simulink model "robo_stix_fn"  (Simulink 7.1)
settings: Solver=FixedStepDiscrete  StartTime=0.0  StopTime=10.0  RelTol=1e-3
settings Model: Creator=jporter  LastModifiedBy=jporter

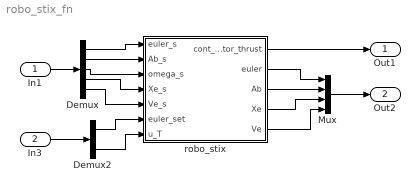
== system robo_stix_fn ==
  In1 : Inport  OutDataType=sfix(16)  OutScaling=2^0
  In3 : Inport  Port=2  OutDataType=sfix(16)  OutScaling=2^0
  Demux : Demux  Outputs=5
  Demux2 : Demux  Outputs=2
  Mux : Mux
  robo_stix : Subsystem
  Out1 : Outport  OutDataType=sfix(16)  OutScaling=2^0
  Out2 : Outport  Port=2  OutDataType=sfix(16)  OutScaling=2^0
  wires:
  Demux/1 -> robo_stix/1(euler_s)
  Demux/2 -> robo_stix/2(Ab_s)
  Demux/3 -> robo_stix/3(omega_s)
  Demux2/1 -> robo_stix/6(euler_set)
  Demux2/2 -> robo_stix/7(u_T)
  In1/1 -> Demux/1
  In3/1 -> Demux2/1
  robo_stix/1(cont_motor_thrust) -> Out1/1
  Mux/1 -> Out2/1
  robo_stix/2(euler) -> Mux/1
  robo_stix/3(Ab) -> Mux/2
  robo_stix/4(Xe) -> Mux/3
  robo_stix/5(Ve) -> Mux/4
  Demux/4 -> robo_stix/4(Xe_s)
  Demux/5 -> robo_stix/5(Ve_s)

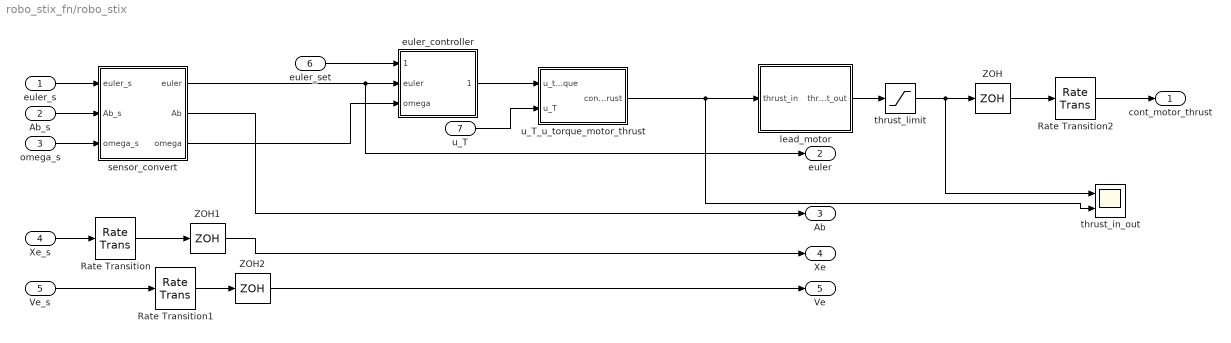
== system robo_stix_fn/robo_stix ==
  euler_s : Inport
  Ab_s : Inport  Port=2
  omega_s : Inport  Port=3
  Xe_s : Inport  Port=4
  Ve_s : Inport  Port=5
  euler_set : Inport  Port=6
  u_T : Inport  Port=7
  Rate Transition : RateTransition
  Rate Transition1 : RateTransition
  Rate Transition2 : RateTransition
  ZOH : ZeroOrderHold
  ZOH1 : ZeroOrderHold
  ZOH2 : ZeroOrderHold
  euler_controller : Subsystem  mask{K=1, K_e=7.5, K_o=.65}
      mask prompts: K "Loop Gain [K]:"; K_e "Euler Gain [K_e]:"; K_o "Omega Gain [K_o]:"
  lead_motor : Subsystem  mask{tau_motor=.1, t_s=.01}
      mask init:
      | a=1/tau_motor;
      | b=pi/t_s;
      | T=t_s;
      | num1=b*(1-exp(-b*T))+a*(b*T-1+exp(-b*T));
      | num2=-b*(1-exp(-b*T))+a*(1-exp(-b*T)-b*T*exp(-b*T));
      | den1=a*b;
      | den2=-a*b*exp(-b*T);
      | num=(b/a)*[num1 num2];
      | den=[den1 den2];
      | Hz=tf(num,den,T);
      | [y,t]=step(Hz);
      | num=(1/y(length(y)))*num;
      | %Hz=(1/y(length(y)))*Hz
      | %bode(Hz);
  sensor_convert : Subsystem  mask{a_g_s=7000, g_g_s=8500}
      mask prompts: a_g_s "AccelGainScale[a_g_s]:"; g_g_s "GyroGainScale[g_g_s]:"
  thrust_in_out : Scope  NumInputPorts=2
      settings: YMin=-5~-5  YMax=5~5  SaveName=ScopeData5
  thrust_limit : Saturate  UpperLimit=10*ones(1,4)  LowerLimit=0*ones(1,4)  OutDataType=sfix(16)  OutScaling=2^0
  u_T_u_torque_motor_thrust : Subsystem  mask{dx=.3048, K_torque=.47}
      mask prompts: dx "X distance of motor from CG [dx](meters):"; K_torque "Ktorque [K_torque]:"
      mask init:
      | M=[0 -dx 0 dx;
      |    dx 0 -dx 0;
      |    -K_torque K_torque -K_torque K_torque;
      |    1 1 1 1];
      | Mi=inv(M);
  cont_motor_thrust : Outport
  euler : Outport  Port=2
  Ab : Outport  Port=3
  Xe : Outport  Port=4
  Ve : Outport  Port=5
  wires:
  euler_s/1 -> sensor_convert/1(euler_s)
  ZOH/1 -> Rate Transition2/1
  Ab_s/1 -> sensor_convert/2(Ab_s)
  omega_s/1 -> sensor_convert/3(omega_s)
  sensor_convert/1(euler) -> euler_controller/2(euler), euler/1
  euler_set/1 -> euler_controller/1(euler_set)
  sensor_convert/3(omega) -> euler_controller/3(omega)
  u_T/1 -> u_T_u_torque_motor_thrust/2(u_T)
  Xe_s/1 -> Rate Transition/1
  Ve_s/1 -> Rate Transition1/1
  euler_controller/1(u_torque) -> u_T_u_torque_motor_thrust/1(u_torque)
  sensor_convert/2(Ab) -> Ab/1
  ZOH1/1 -> Xe/1
  ZOH2/1 -> Ve/1
  Rate Transition/1 -> ZOH1/1
  Rate Transition1/1 -> ZOH2/1
  Rate Transition2/1 -> cont_motor_thrust/1
  u_T_u_torque_motor_thrust/1(cont_motor_thrust) -> lead_motor/1(thrust_in), thrust_in_out/2
  thrust_limit/1 -> ZOH/1, thrust_in_out/1
  lead_motor/1(thrust_out) -> thrust_limit/1

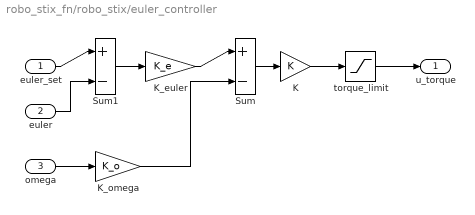
== system robo_stix_fn/robo_stix/euler_controller ==
  euler_set : Inport
  euler : Inport  Port=2
  omega : Inport  Port=3
  K : Gain  Gain=K  ParameterDataType=sfix(16)  ParameterScaling=2^0  OutDataType=sfix(16)  OutScaling=2^0
  K_euler : Gain  Gain=K_e  ParameterDataType=sfix(16)  ParameterScaling=2^0  OutDataType=sfix(16)  OutScaling=2^0
  K_omega : Gain  Gain=K_o  ParameterDataType=sfix(16)  ParameterScaling=2^0  OutDataType=sfix(16)  OutScaling=2^0
  Sum : Sum  Inputs=|+-  OutDataType=sfix(16)  OutScaling=2^0
  Sum1 : Sum  Inputs=|+-  OutDataType=sfix(16)  OutScaling=2^0
  torque_limit : Saturate  UpperLimit=9.8*.3048*ones(1,3)  LowerLimit=-9.8*.3048*ones(1,3)  OutDataType=sfix(16)  OutScaling=2^0
  u_torque : Outport
  wires:
  omega/1 -> K_omega/1
  K/1 -> torque_limit/1
  Sum/1 -> K/1
  K_omega/1 -> Sum/2
  euler_set/1 -> Sum1/1
  Sum1/1 -> K_euler/1
  euler/1 -> Sum1/2
  K_euler/1 -> Sum/1
  torque_limit/1 -> u_torque/1

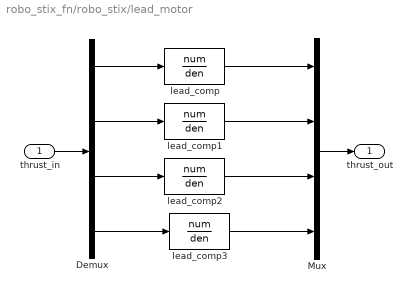
== system robo_stix_fn/robo_stix/lead_motor ==
  thrust_in : Inport
  Demux : Demux
  Mux : Mux
  lead_comp{,1..3} (4 alike) : DiscreteTransferFcn  Numerator=num  Denominator=den  SampleTime=-1
  thrust_out : Outport
  wires:
  thrust_in/1 -> Demux/1
  Mux/1 -> thrust_out/1
  Demux/1 -> lead_comp/1
  lead_comp/1 -> Mux/1
  Demux/2 -> lead_comp1/1
  lead_comp1/1 -> Mux/2
  Demux/3 -> lead_comp2/1
  lead_comp2/1 -> Mux/3
  Demux/4 -> lead_comp3/1
  lead_comp3/1 -> Mux/4

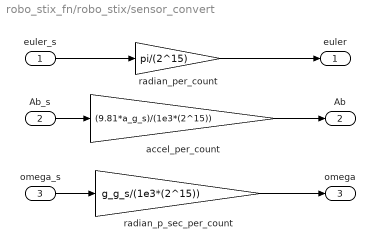
== system robo_stix_fn/robo_stix/sensor_convert ==
  euler_s : Inport
  Ab_s : Inport  Port=2
  omega_s : Inport  Port=3
  accel_per_count : Gain  Gain=(9.81*a_g_s)/(1e3*(2^15))  ParameterDataType=sfix(16)  ParameterScaling=2^0  OutDataType=sfix(16)  OutScaling=2^0
  radian_p_sec_per_count : Gain  Gain=g_g_s/(1e3*(2^15))  ParameterDataType=sfix(16)  ParameterScaling=2^0  OutDataType=sfix(16)  OutScaling=2^0
  radian_per_count : Gain  Gain=pi/(2^15)  ParameterDataType=sfix(16)  ParameterScaling=2^0  OutDataType=sfix(16)  OutScaling=2^0
  euler : Outport
  Ab : Outport  Port=2
  omega : Outport  Port=3
  wires:
  euler_s/1 -> radian_per_count/1
  radian_per_count/1 -> euler/1
  Ab_s/1 -> accel_per_count/1
  accel_per_count/1 -> Ab/1
  omega_s/1 -> radian_p_sec_per_count/1
  radian_p_sec_per_count/1 -> omega/1

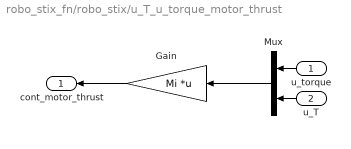
== system robo_stix_fn/robo_stix/u_T_u_torque_motor_thrust ==
  u_torque : Inport  Orientation=left
  u_T : Inport  Orientation=left  Port=2
  Gain : Gain  Orientation=left  Gain=Mi  Multiplication=Matrix(K*u)  ParameterDataType=sfix(16)  ParameterScaling=2^0  OutDataType=sfix(16)  OutScaling=2^0
  Mux : Mux  Orientation=left  Inputs=2
  cont_motor_thrust : Outport  Orientation=left
  wires:
  u_torque/1 -> Mux/1
  Mux/1 -> Gain/1
  u_T/1 -> Mux/2
  Gain/1 -> cont_motor_thrust/1
